simulink model "PLC_SEA"  (R2021a)
settings: Solver=VariableStepAuto  StartTime=0.0  StopTime=10.0  RelTol=1e-3
settings Model: Creator=ShiftSupr  LastModifiedBy=ShiftSupr

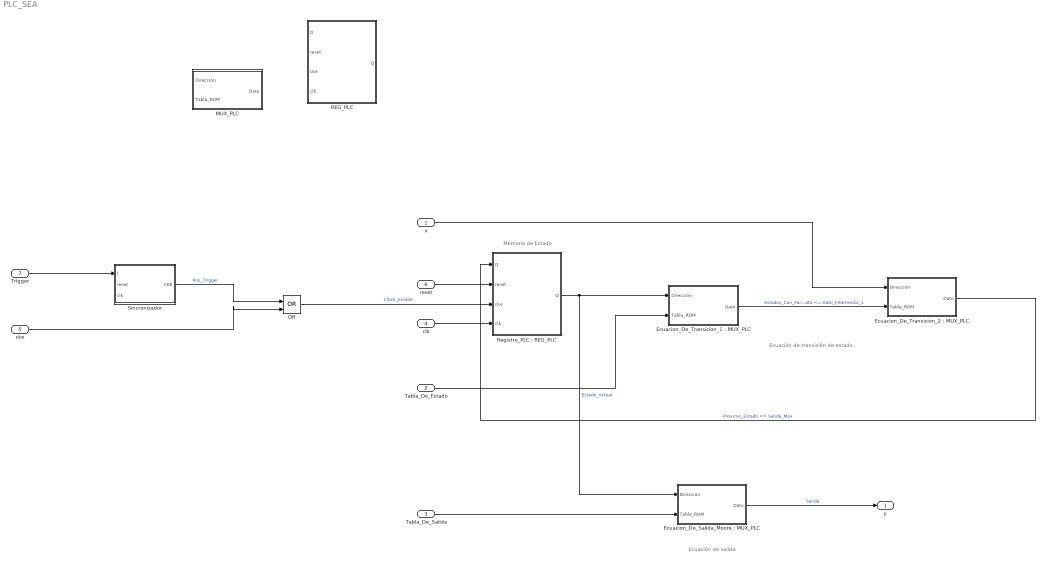
== system PLC_SEA ==
  note: Memoria de Estado
  note: Ecuación de salida
  note: Ecuación de transición de estado
  x : Inport
  Tabla_De_Estado : Inport  Port=2
  Tabla_De_Salida : Inport  Port=3
  clk : Inport  Port=4
  cke : Inport  Port=5
  reset : Inport  Port=6
  Trigger : Inport  Port=7
  "Ecuacion_De_Salida_Moore : MUX_PLC" : Subsystem
  "Ecuacion_De_Transicion_1 : MUX_PLC" : Subsystem
  "Ecuacion_De_Transicion_2 : MUX_PLC" : Subsystem
  MUX_PLC : Subsystem
  OR : Logic  Operator=OR  IconShape=distinctive  AllPortsSameDT=off  OutDataTypeStr=boolean
  REG_PLC : Subsystem
  "Registro_PLC : REG_PLC" : Subsystem
  Sincronizador : Subsystem
  y : Outport
  wires:
  Trigger/1 -> Sincronizador/1(I)
  Sincronizador/1(CKE) -> OR/1  "Pos_Trigger"
  cke/1 -> OR/2
  "Registro_PLC : REG_PLC"/1(Q) -> "Ecuacion_De_Salida_Moore : MUX_PLC"/1(Dirección), "Ecuacion_De_Transicion_1 : MUX_PLC"/1(Dirección)  "Estado_Actual"
  "Ecuacion_De_Transicion_1 : MUX_PLC"/1(Dato) -> "Ecuacion_De_Transicion_2 : MUX_PLC"/2(Tabla_ROM)  "Estados_Con_Formato <= Dato_Intermedio_1"
  Tabla_De_Estado/1 -> "Ecuacion_De_Transicion_1 : MUX_PLC"/2(Tabla_ROM)
  x/1 -> "Ecuacion_De_Transicion_2 : MUX_PLC"/1(Dirección)
  "Ecuacion_De_Transicion_2 : MUX_PLC"/1(Dato) -> "Registro_PLC : REG_PLC"/1(D)  "Proximo_Estado <= Salida_Mux"
  "Ecuacion_De_Salida_Moore : MUX_PLC"/1(Dato) -> y/1  "Salida"
  Tabla_De_Salida/1 -> "Ecuacion_De_Salida_Moore : MUX_PLC"/2(Tabla_ROM)
  OR/1 -> "Registro_PLC : REG_PLC"/3(cke)  "Clock_Enable"
  clk/1 -> "Registro_PLC : REG_PLC"/4(clk)
  reset/1 -> "Registro_PLC : REG_PLC"/2(reset)

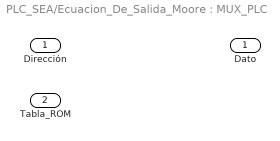
== system PLC_SEA/Ecuacion_De_Salida_Moore : MUX_PLC ==
  Dirección : Inport
  Tabla_ROM : Inport  Port=2
  Dato : Outport

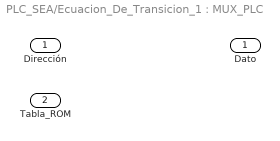
== system PLC_SEA/Ecuacion_De_Transicion_1 : MUX_PLC ==
  Dirección : Inport
  Tabla_ROM : Inport  Port=2
  Dato : Outport

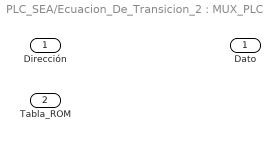
== system PLC_SEA/Ecuacion_De_Transicion_2 : MUX_PLC ==
  Dirección : Inport
  Tabla_ROM : Inport  Port=2
  Dato : Outport

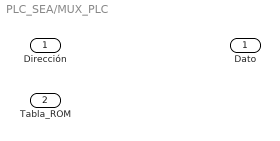
== system PLC_SEA/MUX_PLC ==
  Dirección : Inport
  Tabla_ROM : Inport  Port=2
  Dato : Outport

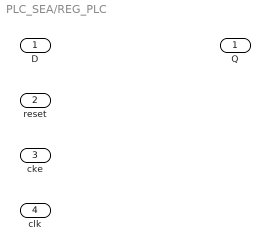
== system PLC_SEA/REG_PLC ==
  D : Inport
  reset : Inport  Port=2
  cke : Inport  Port=3
  clk : Inport  Port=4
  Q : Outport

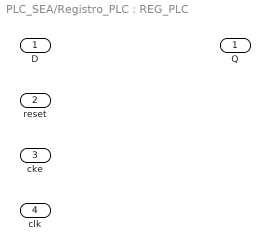
== system PLC_SEA/Registro_PLC : REG_PLC ==
  D : Inport
  reset : Inport  Port=2
  cke : Inport  Port=3
  clk : Inport  Port=4
  Q : Outport

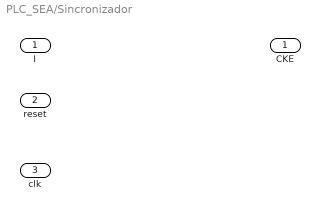
== system PLC_SEA/Sincronizador ==
  I : Inport
  reset : Inport  Port=2
  clk : Inport  Port=3
  CKE : Outport
